simulink model "simulink_carlos_2_4_ziegler"  (R2024b)
settings: Solver=FixedStepAuto  StartTime=0.0  StopTime=20  FixedStep=1e-4  RelTol=1e-3
model workspace (MAT data in the model file):
  C2 = Simulink.Parameter
  C2.Value = 1e-07
  C2.Complexity = 'real'
  C2.Dimensions = [1 1]
  C2.DataType = 'auto'
  C2.DocUnits = 'F'
  C3 = 1e-07
  Jl = 5e-05
  Jm = 5e-05
  La = Simulink.Parameter
  La.Value = 0.05
  La.Complexity = 'real'
  La.Dimensions = [1 1]
  La.DataType = 'auto'
  R11 = 10000
  R2 = 10000
  R3 = 10000
  R4 = 10000
  R5 = 10000
  R6 = 10000
  R7 = 100000
  R8 = 10000
  RV2 = 108000
  RV3 = 121000000
  RV4 = 41255
  Ra = 12
  kt = 0.0205
  kw = 0.0059880239521
  n = Simulink.Parameter
  n.Value = 0.0208333333333
  n.Complexity = 'real'
  n.Dimensions = [1 1]
  n.DataType = 'auto'
values from neighbouring files (symbols this model uses):
  C2 = pid(Kp_zieglerpi,Ki_ziegler)    [practica2_pid_carlos.m]
libraries: fl_lib x10, simulink_extras x2, nesl_utility x2, slpidlib x1
settings Model: Creator=Carlos  LastModifiedBy=carlos
settings HardwareCC: ProdBitPerLong=64  ProdHWDeviceType=Intel->x86-64 (Linux 64)

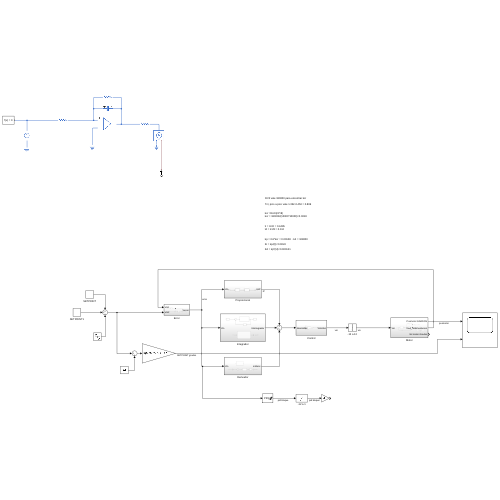
[thumbnail: Simulink's stored preview of the top-level diagram]
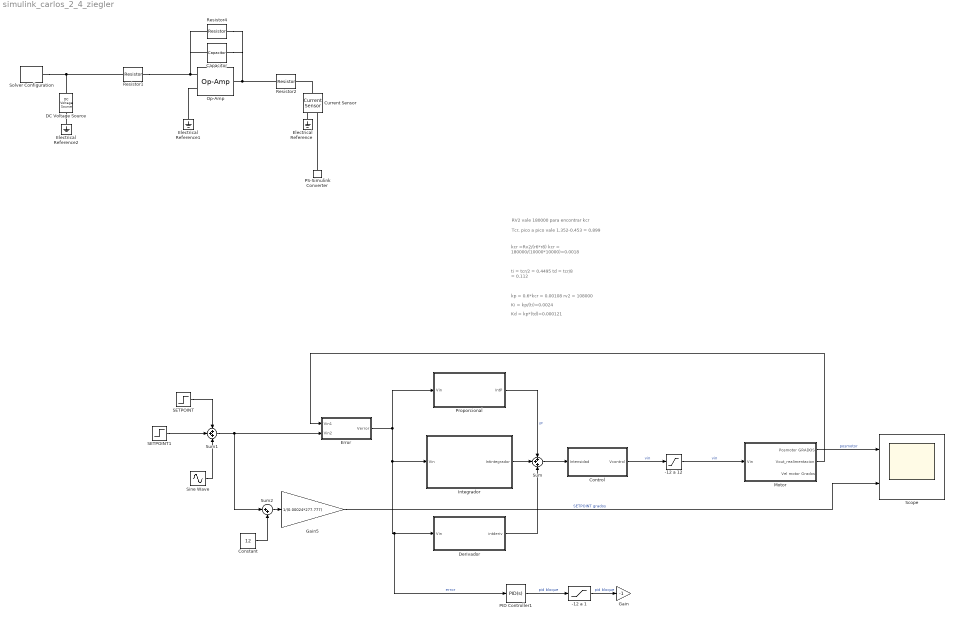
== system simulink_carlos_2_4_ziegler ==
  note: kp = 0.6*kcr = 0.00108 rv2 = 108000
  note: kcr =Rv2/(r6*r8)
      | kcr = 180000/(10000*10000)=0.0018
  note: ti = tcr/2 = 0.4495
      | td = tcr/8 = 0.112
  note: Ki = kp/(ti)=0.0024
  note: Tcr, pico a pico vale 1.352-0.453 = 0.899
  note: RV2 vale 180000 para encontrar kcr
  note: Kd = kp*(td)=0.000121
  -12 a 1 : Saturate  UpperLimit=12  LowerLimit=-12
  -12 a 12 : Saturate  UpperLimit=12  LowerLimit=-12
  Capacitor : fl_lib/Electrical/Electrical Elements/Capacitor  c=C2 F  r=1e-6 Ohm  g=0 1/Ohm  i_specify=off  i_priority=None  i=0 A  i_nominal_specify=off  i_nominal_value=1  i_nominal_unit=A  v_specify=off  v_priority=None  v=0 V  v_nominal_specify=off  v_nominal_value=1  v_nominal_unit=V  vc_specify=off  vc_priority=High  vc=0 V  vc_nominal_specify=off  vc_nominal_value=1  vc_nominal_unit=V
  Constant : Constant  Value=12
  Control : Subsystem
  Current Sensor : fl_lib/Electrical/Electrical Sensors/Current Sensor
  DC Voltage Source : fl_lib/Electrical/Electrical Sources/DC Voltage Source  v0=8 V
  Derivador : Subsystem
  Electrical Reference : fl_lib/Electrical/Electrical Elements/Electrical Reference
  Electrical Reference1 : fl_lib/Electrical/Electrical Elements/Electrical Reference
  Electrical Reference2 : fl_lib/Electrical/Electrical Elements/Electrical Reference
  Error : Subsystem
  Gain : Gain  Gain=-1
  Gain5 : Gain  Gain=1/(0.00024*277.777)
  Integrador : Subsystem
  Motor : Subsystem
  Op-Amp : fl_lib/Electrical/Electrical Elements/Op-Amp  outI_specify=off  outI_priority=None  outI=0 A  outI_nominal_specify=off  outI_nominal_value=1  outI_nominal_unit=A
  PID Controller1 : slpidlib/PID Controller  Controller=PID  Form=Ideal  TimeDomain=Continuous-time  UseExternalTs=off  SampleTime=-1  IntegratorMethod=Forward Euler  FilterMethod=Forward Euler  ControllerParametersSource=internal  P=1.19656996243384  I=0.217709378370413  UseKiTs=off  D=0.907329336894528  UseExternalDerivativeSource=off  N=8.67199300276142  UseFilter=on  TunerSelectOption=Transfer Function Based (PID Tuner App)  InitialConditionSource=internal  InitialConditionForIntegrator=0  InitialConditionForFilter=0  DifferentiatorICPrevScaledInput=0  ExternalReset=none  TrackingMode=off  Kt=1  LimitOutput=on  SatLimitsSource=internal  UpperSaturationLimit=12  LowerSaturationLimit=-12  LinearizeAsGain=on  AntiWindupMode=none  Kb=1  LimitIntegrator=off  UpperIntegratorSaturationLimit=inf  LowerIntegratorSaturationLimit=-inf  SaturateOnIntegerOverflow=on  POutMin=[]  POutMax=[]  IOutMin=[]  IOutMax=[]  DOutMin=[]  DOutMax=[]  NOutMin=[]  NOutMax=[]  SumOutMin=[]  SumOutMax=[]  SaturationOutMin=[]  SaturationOutMax=[]  PParamMin=[]  PParamMax=[]  IParamMin=[]  IParamMax=[]  DParamMin=[]  DParamMax=[]  NParamMin=[]  NParamMax=[]  KbParamMin=[]  KbParamMax=[]  KtParamMin=[]  KtParamMax=[]  KbOutMin=[]  KbOutMax=[]  KtOutMin=[]  KtOutMax=[]  IntegratorOutMin=[]  IntegratorOutMax=[]  FilterOutMin=[]  FilterOutMax=[]  SumI1OutMin=[]  SumI1OutMax=[]  SumI2OutMin=[]  SumI2OutMax=[]  SumI3OutMin=[]  SumI3OutMax=[]  SumI4OutMin=[]  SumI4OutMax=[]  SumDOutMin=[]  SumDOutMax=[]  DifferentiatorOutMin=[]  DifferentiatorOutMax=[]  FilterDiffOutCoefMin=[]  FilterDiffOutCoefMax=[]  ReciprocalOutMin=[]  ReciprocalOutMax=[]  SumDenOutMin=[]  SumDenOutMax=[]  SumNumOutMin=[]  SumNumOutMax=[]  DivideOutMin=[]  DivideOutMax=[]  UdiffTsProdOutMin=[]  UdiffTsProdOutMax=[]  NTsProdOutMin=[]  NTsProdOutMax=[]  UintegralTsProdOutMin=[]  UintegralTsProdOutMax=[]  UngainTsProdOutMin=[]  UngainTsProdOutMax=[]  ClampingZeroOutDataTypeStr=Inherit: Inherit via back propagation  ClampingZeroOutMin=[]  ClampingZeroOutMax=[]  FilterDenConstantOutDataTypeStr=Inherit: Inherit via back propagation  FilterDenConstantOutMin=[]  FilterDenConstantOutMax=[]  PCopyOutDataTypeStr=Inherit: Inherit via back propagation  PCopyOutMin=[]  PCopyOutMax=[]  NCopyOutDataTypeStr=Inherit: Inherit via back propagation  NCopyOutMin=[]  NCopyOutMax=[]  IntegratorContinuousStateAttributes=''  IntegratorStateMustResolveToSignalObject=off  IntegratorRTWStateStorageClass=Auto  FilterContinuousStateAttributes=''  FilterStateMustResolveToSignalObject=off  FilterRTWStateStorageClass=Auto  ParallelPVariant=InternalParameters  IdealPVariant=Disabled  IVariant=InternalParameters  DVariant=InternalParameters  IntegratorVariant=Continuous  SatVariant=Disabled  AWVariant=Passthrough  PCopyVariant=Disabled  TRVariant=Disabled  FdbkBlocksVariant=Forward  IdealPFdbkVariant=Disabled  SatFdbkVariant=Disabled  DerivativeFilterVariant=ContFilter  NVariant=InternalParameters  NCopyVariant=Disabled  FilterICVariant=InternalICsFilter  IntegratorICVariant=InternalICs  ExternalResetVariant=Disabled  TRSumVariant=Passthrough  SumFdbkVariant=Disabled  SumVariant=Sum_PID  TsampFilterVariant=InternalTs  TsampNgainVariant=Passthrough  TsampIntegralVariant=Passthrough  ExternalSaturationOutDataTypeStr=Inherit: Same as second input  DerivativeSourceVariant=ErrorSignal  PreIntVariant=InternalPreInt
  PS-Simulink Converter : nesl_utility/PS-Simulink Converter  PhysicalDomain=network_engine_domain  SubClassName=ps_output  LeftPortType=input  RightPortType=output  PseudoPeriodic=off  Frequencies=[]  VectorFormat=inherit  Unit=inherit  AffineConversion=off
  Proporcional : Subsystem
  Resistor1 : fl_lib/Electrical/Electrical Elements/Resistor  R=RV4 Ohm  i_specify=off  i_priority=None  i=0 A  i_nominal_specify=off  i_nominal_value=1  i_nominal_unit=A  v_specify=off  v_priority=None  v=0 V  v_nominal_specify=off  v_nominal_value=1  v_nominal_unit=V
  Resistor2 : fl_lib/Electrical/Electrical Elements/Resistor  R=R8 Ohm  i_specify=off  i_priority=None  i=0 A  i_nominal_specify=off  i_nominal_value=1  i_nominal_unit=A  v_specify=off  v_priority=None  v=0 V  v_nominal_specify=off  v_nominal_value=1  v_nominal_unit=V
  Resistor4 : fl_lib/Electrical/Electrical Elements/Resistor  R=R7 Ohm  i_specify=off  i_priority=None  i=0 A  i_nominal_specify=off  i_nominal_value=1  i_nominal_unit=A  v_specify=off  v_priority=None  v=0 V  v_nominal_specify=off  v_nominal_value=1  v_nominal_unit=V
  SETPOINT : Step  Time=0  After=6  SampleTime=0
  SETPOINT1 : Step  Time=10  After=-10  SampleTime=0
  Scope : Scope  NumInputPorts=2
  Sine Wave : Sin  Amplitude=6  Frequency=0.5  SampleTime=0
  Solver Configuration : nesl_utility/Solver Configuration  PhysicalDomain=network_engine_domain  SubClassName=solver  LeftPortType=input  RightPortType=generic  Tones=[]  Harmonics=[]  SimulateNoise=off  Profile=off  UseLocalSampling=off  EnableSwitchedLinearOptims=on  FrequencyDomain=off  UseCCode=off  RelTol=0.001  AbsTol=0.001  MinStep=1e-09  ToWorkspace=off  RevertToSquareIcSolve=off  NumHomotopyIterations=100  PhasorMode=off  PhasorModeNumHarmonics=1  ConsistencySolver=NEWTON_XTOL_AFTER_FTOL  IndexReductionMethod=DerivativeReplacement  DoDC=off  ResidualTolerance=1e-09  ConsistencyTolSource=GLOBAL  ConsistencyAbsTol=0.001  ConsistencyRelTol=0.001  ConsistencyTolFactor=0.001  UseLocalSolver=off  LocalSolverChoice=NE_BACKWARD_EULER_ADVANCER  ResolveIndetEquations=on  FunctionEvalNumThread=1  LocalSolverSampleTime=0.001  DoFixedCost=off  MaxNonlinIter=3  MaxModeIter=2  ComputeImpulses=off  ImpulseIterations=2  LinearAlgebra=auto  LinearAlgebraNumThread=0  EquationFormulation=NE_TIME_EF  DelaysMemoryBudget=1024  AutomaticFiltering=on  FilteringTimeConstant=0.001  PartitionStorageMethod=AS_NEEDED  PartitionMemoryBudget=1024  PartitionMethod=ROBUST  MultibodyUseLocalSolver=off  MultibodyLocalSolverChoice=ODE1  MultibodyLocalSolverSampleTime=0.001
  Sum : Sum  Inputs=+++
  Sum1 : Sum  Inputs=+++
  Sum2 : Sum  Inputs=|++
  wires:
  Error/1(Verror) -> Proporcional/1(Vin), Integrador/1(Vin), PID Controller1/1, Derivador/1(Vin)  "error"
  Motor/2(Vout_realimentacion) -> Error/1(Vin1)
  Sum1/1 -> Sum2/1, Error/2(Vin2)
  Motor/1(Posmotor GRADOS) -> Scope/1  "posmotor"
  Constant/1 -> Sum2/2
  Sum2/1 -> Gain5/1
  Sum/1 -> Control/1(Intensidad)
  Gain5/1 -> Scope/2  "SETPOINT grados"
  SETPOINT/1 -> Sum1/1
  Control/1(Vcontrol) -> -12 a 12/1  "vin"
  PID Controller1/1 -> -12 a 1/1  "pid bloque"
  Proporcional/1(IntP) -> Sum/1  "iP"
  SETPOINT1/1 -> Sum1/2
  Integrador/1(Intintegrador) -> Sum/2
  Derivador/1(intderiv) -> Sum/3
  -12 a 1/1 -> Gain/1  "pid bloque"
  Sine Wave/1 -> Sum1/3
  -12 a 12/1 -> Motor/1(Vin)  "vin"
  connections:
  Resistor2/LConn1 -- Capacitor/RConn1 -- Resistor4/RConn1 -- Op-Amp/RConn1
  Solver Configuration/RConn1 -- DC Voltage Source/LConn1 -- Resistor1/LConn1
  PS-Simulink Converter/LConn1 -- Current Sensor/RConn1
  Electrical Reference2/LConn1 -- DC Voltage Source/RConn1
  Resistor1/RConn1 -- Capacitor/LConn1 -- Resistor4/LConn1 -- Op-Amp/LConn1
  Electrical Reference1/LConn1 -- Op-Amp/LConn2
  Current Sensor/LConn1 -- Resistor2/RConn1
  Electrical Reference/LConn1 -- Current Sensor/RConn2

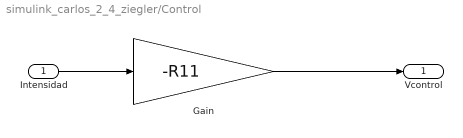
== system simulink_carlos_2_4_ziegler/Control ==
  Intensidad : Inport
  Gain : Gain  Gain=-R11
  Vcontrol : Outport
  wires:
  Intensidad/1 -> Gain/1
  Gain/1 -> Vcontrol/1

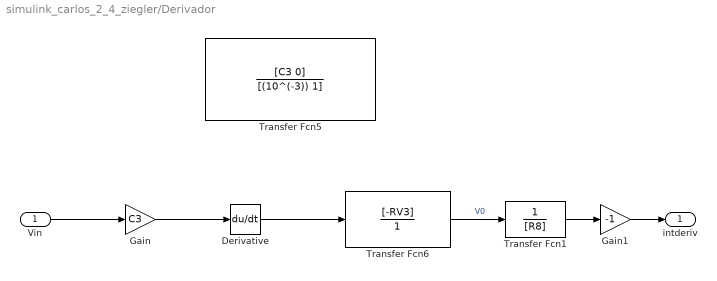
== system simulink_carlos_2_4_ziegler/Derivador ==
  Vin : Inport
  Derivative : Derivative
  Gain : Gain  Gain=C3
  Gain1 : Gain  Gain=-1
  Transfer Fcn1 : TransferFcn  Denominator=[R8]
  Transfer Fcn5 : TransferFcn  Numerator=[C3 0]  Denominator=[(10^(-3)) 1]
  Transfer Fcn6 : TransferFcn  Numerator=[-RV3]  Denominator=[1]
  intderiv : Outport
  wires:
  Transfer Fcn6/1 -> Transfer Fcn1/1  "V0"
  Derivative/1 -> Transfer Fcn6/1
  Vin/1 -> Gain/1
  Gain/1 -> Derivative/1
  Transfer Fcn1/1 -> Gain1/1
  Gain1/1 -> intderiv/1

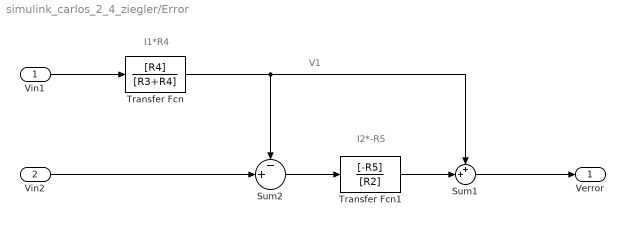
== system simulink_carlos_2_4_ziegler/Error ==
  note: I2*-R5
  note: V1
  note: I1*R4
  Vin1 : Inport
  Vin2 : Inport  Port=2
  Sum1 : Sum  Inputs=++|
  Sum2 : Sum  Inputs=-+|
  Transfer Fcn : TransferFcn  Numerator=[R4]  Denominator=[R3+R4]
  Transfer Fcn1 : TransferFcn  Numerator=[-R5]  Denominator=[R2]
  Verror : Outport
  wires:
  Vin1/1 -> Transfer Fcn/1
  Transfer Fcn/1 -> Sum1/1, Sum2/1
  Vin2/1 -> Sum2/2
  Sum2/1 -> Transfer Fcn1/1
  Transfer Fcn1/1 -> Sum1/2
  Sum1/1 -> Verror/1

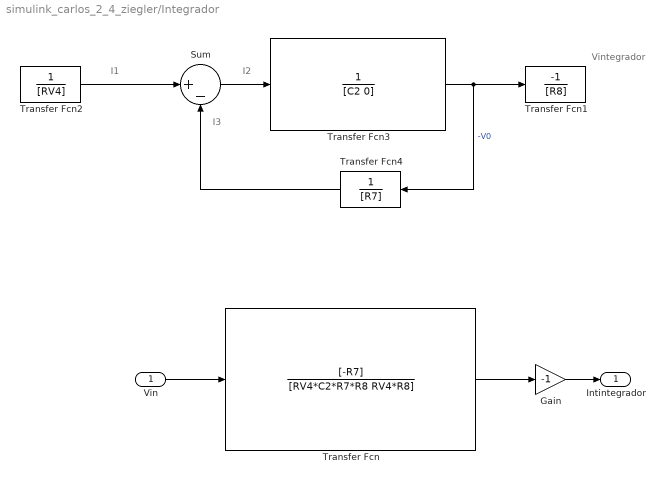
== system simulink_carlos_2_4_ziegler/Integrador ==
  note: I2
  note: I3
  note: I1
  note: Vintegrador
  Vin : Inport
  Gain : Gain  Gain=-1
  Sum : Sum  Inputs=|+-
  Transfer Fcn : TransferFcn  Numerator=[-R7]  Denominator=[RV4*C2*R7*R8 RV4*R8]
  Transfer Fcn1 : TransferFcn  Numerator=[-1]  Denominator=[R8]
  Transfer Fcn2 : TransferFcn  Denominator=[RV4]
  Transfer Fcn3 : TransferFcn  Denominator=[C2 0]
  Transfer Fcn4 : TransferFcn  Denominator=[R7]
  Intintegrador : Outport
  wires:
  Transfer Fcn3/1 -> Transfer Fcn1/1, Transfer Fcn4/1  "-V0"
  Transfer Fcn2/1 -> Sum/1
  Sum/1 -> Transfer Fcn3/1
  Transfer Fcn4/1 -> Sum/2
  Vin/1 -> Transfer Fcn/1
  Transfer Fcn/1 -> Gain/1
  Gain/1 -> Intintegrador/1

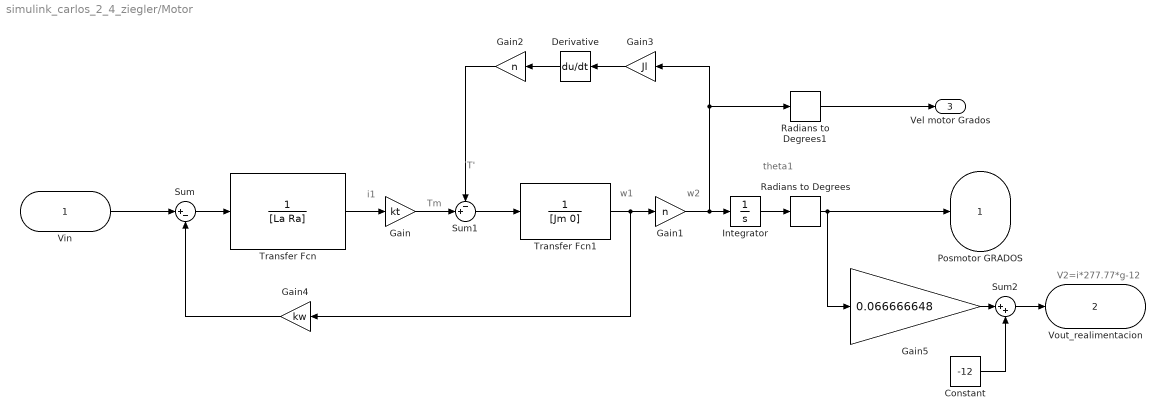
== system simulink_carlos_2_4_ziegler/Motor ==
  note: V2=i*277.77*g-12
  note: T'
  note: theta1
  note: w1
  note: w2
  note: i1
  note: Tm
  Vin : Inport
  Constant : Constant  Value=-12
  Derivative : Derivative
  Gain : Gain  Gain=kt
  Gain1 : Gain  Gain=n
  Gain2 : Gain  Gain=n
  Gain3 : Gain  Gain=Jl
  Gain4 : Gain  Gain=kw
  Gain5 : Gain  Gain=0.066666648
  Integrator : Integrator
  Radians to Degrees : simulink_extras/Transformations/Radians to Degrees
  Radians to Degrees1 : simulink_extras/Transformations/Radians to Degrees
  Sum : Sum  Inputs=|+-
  Sum1 : Sum  Inputs=-+|
  Sum2 : Sum  Inputs=|++
  Transfer Fcn : TransferFcn  Denominator=[La Ra]
  Transfer Fcn1 : TransferFcn  Denominator=[Jm 0]
  Posmotor GRADOS : Outport
  Vout_realimentacion : Outport  Port=2
  Vel motor Grados : Outport  Port=3
  wires:
  Transfer Fcn/1 -> Gain/1
  Sum/1 -> Transfer Fcn/1
  Gain/1 -> Sum1/2
  Sum1/1 -> Transfer Fcn1/1
  Transfer Fcn1/1 -> Gain4/1, Gain1/1
  Integrator/1 -> Radians to Degrees/1
  Gain1/1 -> Radians to Degrees1/1, Gain3/1, Integrator/1
  Derivative/1 -> Gain2/1
  Gain3/1 -> Derivative/1
  Vin/1 -> Sum/1
  Gain4/1 -> Sum/2
  Gain5/1 -> Sum2/1
  Sum2/1 -> Vout_realimentacion/1
  Constant/1 -> Sum2/2
  Radians to Degrees/1 -> Gain5/1, Posmotor GRADOS/1
  Radians to Degrees1/1 -> Vel motor Grados/1
  Gain2/1 -> Sum1/1

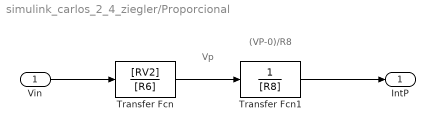
== system simulink_carlos_2_4_ziegler/Proporcional ==
  note: (VP-0)/R8
  note: Vp
  Vin : Inport
  Transfer Fcn : TransferFcn  Numerator=[RV2]  Denominator=[R6]
  Transfer Fcn1 : TransferFcn  Denominator=[R8]
  IntP : Outport
  wires:
  Vin/1 -> Transfer Fcn/1
  Transfer Fcn/1 -> Transfer Fcn1/1
  Transfer Fcn1/1 -> IntP/1
